simulink model "mod11"  (Simulink 8.9)
settings: Solver=ode45  StartTime=0.0  StopTime=10  RelTol=1e-3  AbsTol=1e-6
values from neighbouring files (symbols this model uses):
  B = 0.8    [par11.m]
  J = 0.08    [par11.m]
  Kp = 10    [par11.m]
  Kt = 0.5    [par11.m]
  Kv = 1.0    (= 1)    [par11.m]
  La = 0.004    [par11.m]
  Ra = 0.4    [par11.m]
  Theta0 = 0    [par11.m]
  TL = 0    [par11.m]
settings Model: Creator=anderalb  LastModifiedBy=bruker  ExtModeTrigMode=oneshot  ExtModeArmWhenConnect=off
settings DataIOCC: LimitDataPoints=off
settings OptimizationCC: BlockReduction=off  BooleanDataType=off
settings DebuggingCC: SaveWithParameterizedLinksMsg=none  SignalResolutionControl=TryResolveAllWithWarning  MultiTaskDSMMsg=warning  MultiTaskCondExecSysMsg=none  FcnCallInpInsideContextMsg=error
settings HardwareCC: TargetUnknown=on

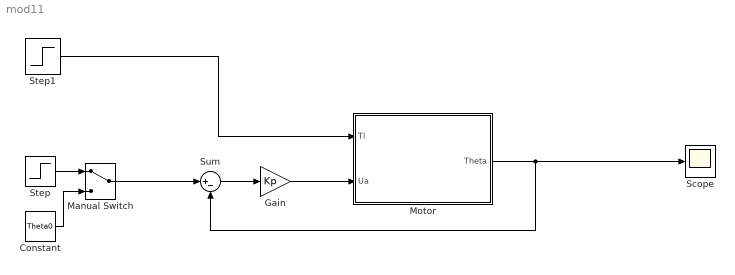
== system mod11 ==
  Constant : Constant  Value=Theta0
  Gain : Gain  Gain=Kp
  Manual Switch : ManualSwitch
  Motor : Subsystem
  Scope : Scope
  Step : Step  SampleTime=0
  Step1 : Step  After=TL  SampleTime=0
  Sum : Sum  Inputs=|+-
  wires:
  Step1/1 -> Motor/1(Tl)
  Motor/1(Theta) -> Scope/1, Sum/2
  Gain/1 -> Motor/2(Ua)
  Sum/1 -> Gain/1
  Step/1 -> Manual Switch/1
  Manual Switch/1 -> Sum/1
  Constant/1 -> Manual Switch/2

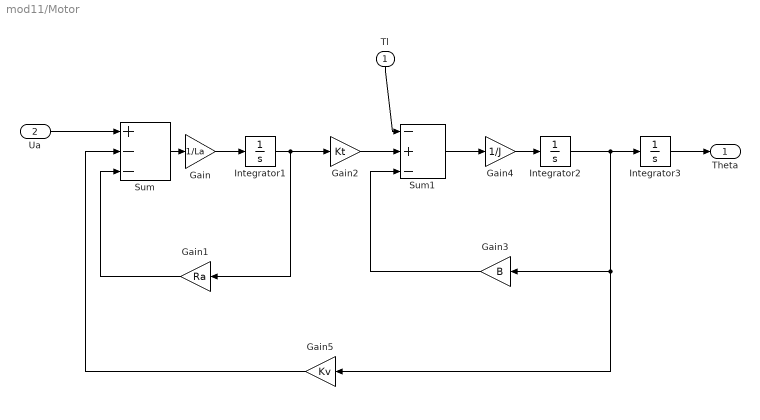
== system mod11/Motor ==
  Tl : Inport
  Ua : Inport  Port=2
  Gain : Gain  Gain=1/La  SaturateOnIntegerOverflow=on  OutDataTypeStr=Inherit: Same as input  ParamDataTypeStr=Inherit: Same as input
  Gain1 : Gain  Gain=Ra  SaturateOnIntegerOverflow=on  OutDataTypeStr=Inherit: Same as input  ParamDataTypeStr=Inherit: Same as input
  Gain2 : Gain  Gain=Kt  SaturateOnIntegerOverflow=on  OutDataTypeStr=Inherit: Same as input  ParamDataTypeStr=Inherit: Same as input
  Gain3 : Gain  Gain=B  SaturateOnIntegerOverflow=on  OutDataTypeStr=Inherit: Same as input  ParamDataTypeStr=Inherit: Same as input
  Gain4 : Gain  Gain=1/J  SaturateOnIntegerOverflow=on  OutDataTypeStr=Inherit: Same as input  ParamDataTypeStr=Inherit: Same as input
  Gain5 : Gain  Gain=Kv  SaturateOnIntegerOverflow=on  OutDataTypeStr=Inherit: Same as input  ParamDataTypeStr=Inherit: Same as input
  Integrator1 : Integrator
  Integrator2 : Integrator  InitialCondition=200
  Integrator3 : Integrator
  Sum : Sum  Inputs=+--  SaturateOnIntegerOverflow=on  InputSameDT=on  OutDataTypeStr=Inherit: Same as first input
  Sum1 : Sum  Inputs=-+-  SaturateOnIntegerOverflow=on  InputSameDT=on  OutDataTypeStr=Inherit: Same as first input
  Theta : Outport  InitialOutput=0
  wires:
  Integrator3/1 -> Theta/1
  Integrator2/1 -> Gain5/1, Gain3/1, Integrator3/1
  Gain4/1 -> Integrator2/1
  Integrator1/1 -> Gain1/1, Gain2/1
  Gain/1 -> Integrator1/1
  Sum1/1 -> Gain4/1
  Tl/1 -> Sum1/1
  Gain3/1 -> Sum1/3
  Ua/1 -> Sum/1
  Gain5/1 -> Sum/2
  Gain2/1 -> Sum1/2
  Gain1/1 -> Sum/3
  Sum/1 -> Gain/1
